simulink model "sis_com_red_atraso"  (R2020b)
settings: Solver=VariableStepAuto  StartTime=0.0  StopTime=100  MaxStep=1e-2  RelTol=1e-3
libraries: simulink x1
settings Model: Creator=carma  LastModifiedBy=carma

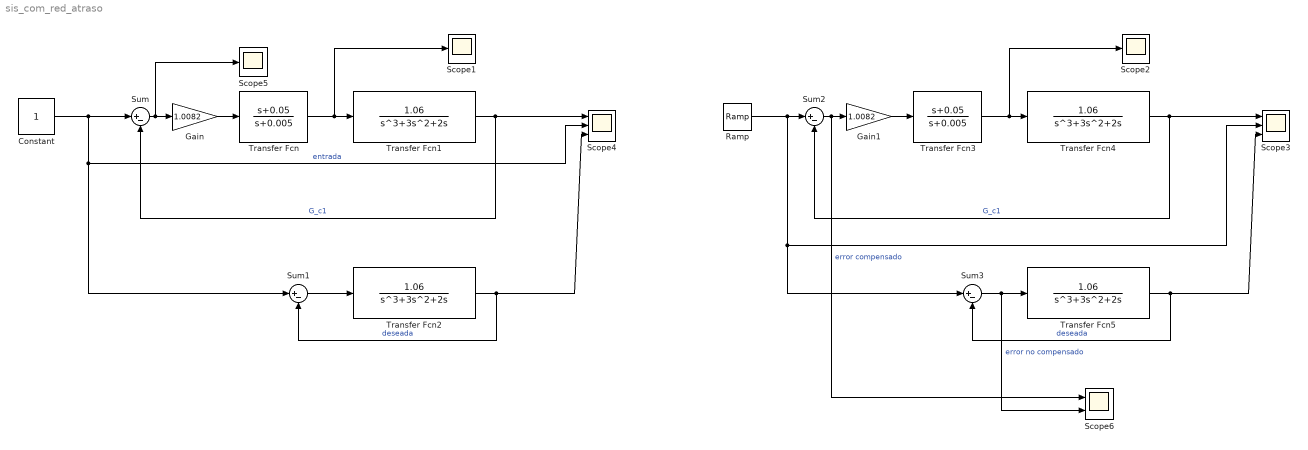
== system sis_com_red_atraso ==
  Constant : Constant  VectorParams1D=off  SampleTime=-1
  Gain : Gain  Gain=1.0082
  Gain1 : Gain  Gain=1.0082
  Ramp : simulink/Sources/Ramp  slope=1  start=0  InitialOutput=0
  Scope1 : Scope
  Scope2 : Scope
  Scope3 : Scope  NumInputPorts=3
  Scope4 : Scope  NumInputPorts=3
  Scope5 : Scope
  Scope6 : Scope  NumInputPorts=2
  Sum{,1..3} (4 alike) : Sum  Inputs=|+-
  Transfer Fcn : TransferFcn  Numerator=[1 0.05]  Denominator=[1 0.005]
  Transfer Fcn{1..2,4..5} (4 alike) : TransferFcn  Numerator=1.06  Denominator=[1 3 2 0]
  Transfer Fcn3 : TransferFcn  Numerator=[1 0.05]  Denominator=[1 0.005]
  wires:
  Constant/1 -> Sum/1, Sum1/1, Scope4/2  "entrada"
  Sum/1 -> Scope5/1, Gain/1
  Gain/1 -> Transfer Fcn/1
  Transfer Fcn/1 -> Scope1/1, Transfer Fcn1/1
  Transfer Fcn1/1 -> Scope4/1, Sum/2  "G_c1"
  Sum1/1 -> Transfer Fcn2/1
  Transfer Fcn2/1 -> Scope4/3, Sum1/2  "deseada"
  Transfer Fcn5/1 -> Scope3/3, Sum3/2  "deseada"
  Transfer Fcn4/1 -> Scope3/1, Sum2/2  "G_c1"
  Gain1/1 -> Transfer Fcn3/1
  Transfer Fcn3/1 -> Scope2/1, Transfer Fcn4/1
  Sum2/1 -> Scope6/1, Gain1/1  "error compensado"
  Ramp/1 -> Sum3/1, Scope3/2, Sum2/1
  Sum3/1 -> Scope6/2, Transfer Fcn5/1  "error no compensado"
